simulink model "Lab1T1"  (R2017b)
settings: Solver=ode45  StartTime=0.0  StopTime=100  RelTol=1e-5
settings Model: Creator=aloisia  LastModifiedBy=aloisia

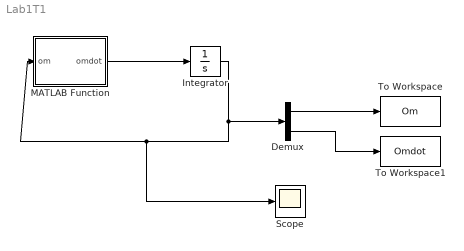
== system Lab1T1 ==
  Demux : Demux  Outputs=2
  Integrator : Integrator  InitialCondition=[0.45;0.52;0.55]
  MATLAB Function : MATLAB Function  TreatAsAtomicUnit=on
  Scope : Scope
  To Workspace : ToWorkspace  VariableName=Om  SaveFormat=Timeseries  SampleTime=-1
  To Workspace1 : ToWorkspace  VariableName=Omdot  SaveFormat=Timeseries  SampleTime=-1
  wires:
  MATLAB Function/1(omdot) -> Integrator/1
  Integrator/1 -> Demux/1, Scope/1, MATLAB Function/1(om)
  Demux/2 -> To Workspace1/1
  Demux/1 -> To Workspace/1

== matlab function Lab1T1/MATLAB Function ==
  data: om input; omdot output
function omdot = Euler_eq(om)

% om = [wx; wy; wz];
Ix = 0.07; %[kgm^2]
Iy = 0.0504; %[kgm^2]
Iz = 0.0109; %[kgm^2]

omdot = zeros(3,1);
omdot(1) = (Iy - Iz)/Ix * om(2)*om(3);
omdot(2) = (Iz - Ix)/Iy * om(1)*om(3);
omdot(3) = (Ix - Iy)/Iz * om(2)*om(1);
